simulink model "gm_SuFrame_Scrambler"  (R2023b)
settings: Solver=VariableStepAuto  StartTime=0.0  StopTime=10000/fs  RelTol=1e-3
undefined symbols (not defined in the file or in its folder): fs, iniStates, n, sourceData
libraries: hdlsllib x5, simulink x4
settings Model: Creator=31651  LastModifiedBy=31651
settings OptimizationCC: BlockReduction=off  ConditionallyExecuteInputs=off
settings DebuggingCC: ArtificialAlgebraicLoopMsg=none  InheritedTsInSrcMsg=none

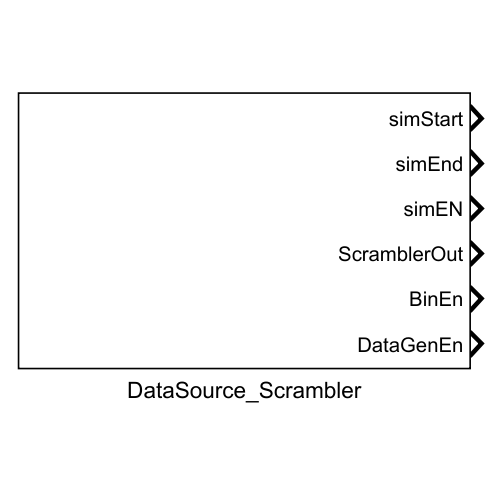
[thumbnail: Simulink's stored preview of the top-level diagram]
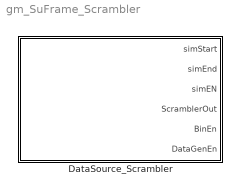
== system gm_SuFrame_Scrambler ==
  DataSource_Scrambler : Subsystem

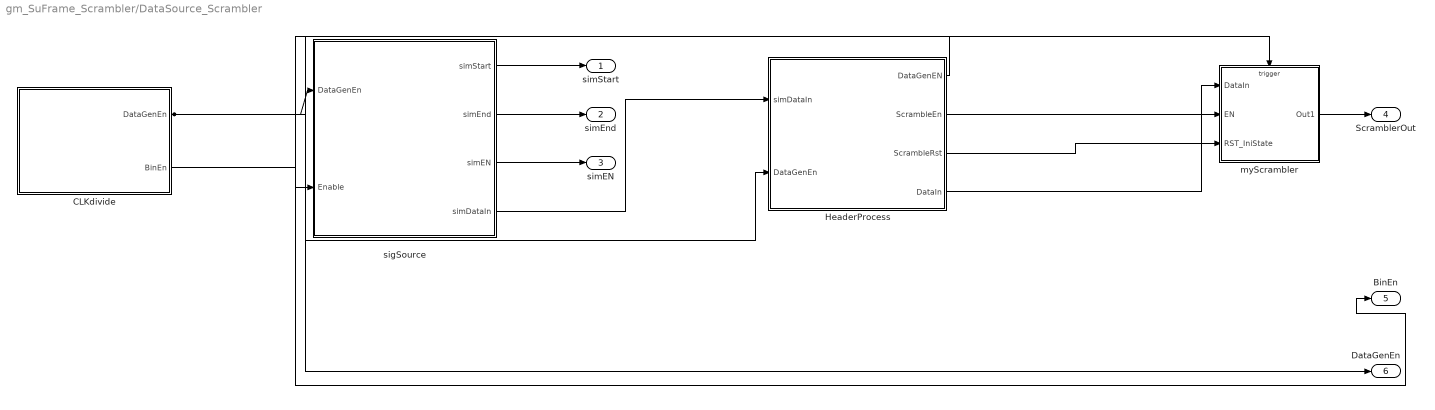
== system gm_SuFrame_Scrambler/DataSource_Scrambler ==
  CLKdivide : Subsystem
  HeaderProcess : Subsystem
  myScrambler : Subsystem
  sigSource : Subsystem
  simStart : Outport  SampleTime=5e-09
  simEnd : Outport  Port=2  SampleTime=5e-09
  simEN : Outport  Port=3  SampleTime=5e-09
  ScramblerOut : Outport  Port=4  SampleTime=5e-09
  BinEn : Outport  Port=5  SampleTime=5e-09  VectorParamsAs1DForOutWhenUnconnected=off
  DataGenEn : Outport  Port=6  SampleTime=5e-09  VectorParamsAs1DForOutWhenUnconnected=off
  wires:
  CLKdivide/1(DataGenEn) -> DataGenEn/1, myScrambler/Trigger, HeaderProcess/2(DataGenEn), sigSource/1(DataGenEn)
  CLKdivide/2(BinEn) -> BinEn/1
  HeaderProcess/2(ScrambleEn) -> myScrambler/2(EN)
  HeaderProcess/3(ScrambleRst) -> myScrambler/3(RST_IniState)
  HeaderProcess/4(DataIn) -> myScrambler/1(DataIn)
  myScrambler/1(Out1) -> ScramblerOut/1
  sigSource/1(simStart) -> simStart/1
  sigSource/2(simEnd) -> simEnd/1
  sigSource/3(simEN) -> simEN/1
  HeaderProcess/1(DataGenEN) -> sigSource/2(Enable)
  sigSource/4(simDataIn) -> HeaderProcess/1(simDataIn)

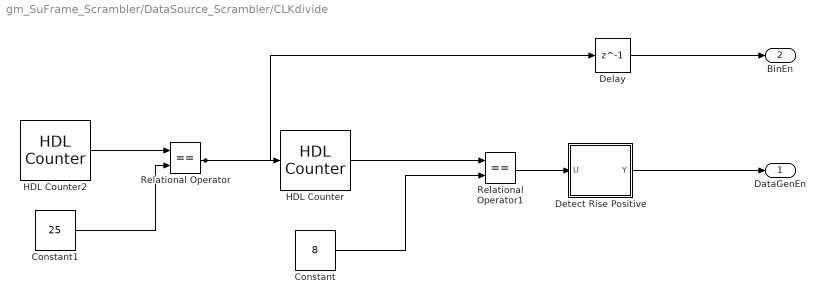
== system gm_SuFrame_Scrambler/DataSource_Scrambler/CLKdivide ==
  Constant : Constant  Value=8  VectorParams1D=off  OutDataTypeStr=uint8  SampleTime=-1
  Constant1 : Constant  Value=25  VectorParams1D=off  OutDataTypeStr=uint8  SampleTime=-1
  Delay : Delay  DelayLength=1
  Detect Rise Positive : Subsystem  mask(Detect Rise Positive){vinit=double(0), InputProcessing=Elements as channels (sample based), OutDataTypeStr=boolean}
      mask prompts: vinit "Simulink:masks:InitialCondition_MP"; InputProcessing "Simulink:masks:InputProcessing_MP"; OutDataTypeStr "Simulink:masks:OutputDataType_MP"
      mask help: Simulink:masks:DetectRisePositive_MD
      mask init:
      | InputProcessing = 'Elements as channels (sample based)';
      | OutDataTypeStr = 'boolean';
      | vinit = double(0);
      mask TypeOptions InputProcessing: Simulink:masks:ColumnsAsChannelsFrameBased | Simulink:masks:ElementsAsChannelsSampleBased
      mask TypeOptions OutDataTypeStr: Simulink:masks:uint8 | Simulink:masks:boolean
      mask Display: fprintf('U > 0\n&  NOT\nU/z > 0')
  HDL Counter : hdlsllib/Sources/HDL Counter  CountType=Count limited  CountInit=1  CountStep=1  CountMax=8  CountFromType=Initial value  CountFrom=1  CountResetPort=off  CountLoadPort=off  CountEnbPort=on  CountDirPort=off  CountHitOutputPort=off  CountDataType=Unsigned  CountWordLen=8  CountFracLen=0  CountSampTime=1
  HDL Counter2 : hdlsllib/Sources/HDL Counter  CountType=Count limited  CountInit=1  CountStep=1  CountMax=25  CountFromType=Initial value  CountFrom=1  CountResetPort=off  CountLoadPort=off  CountEnbPort=off  CountDirPort=off  CountHitOutputPort=off  CountDataType=Unsigned  CountWordLen=8  CountFracLen=0  CountSampTime=1/fs
  Relational Operator : RelationalOperator  Operator===  OutDataTypeStr=boolean  InputSameDT=off
  Relational Operator1 : RelationalOperator  Operator===  OutDataTypeStr=boolean  InputSameDT=off
  DataGenEn : Outport  SampleTime=5e-09  VectorParamsAs1DForOutWhenUnconnected=off
  BinEn : Outport  Port=2  SampleTime=5e-09  VectorParamsAs1DForOutWhenUnconnected=off
  wires:
  Constant/1 -> Relational Operator1/2
  Constant1/1 -> Relational Operator/2
  Delay/1 -> BinEn/1
  Detect Rise Positive/1(Y) -> DataGenEn/1
  HDL Counter/1 -> Relational Operator1/1
  HDL Counter2/1 -> Relational Operator/1
  Relational Operator/1 -> Delay/1, HDL Counter/1
  Relational Operator1/1 -> Detect Rise Positive/1(U)

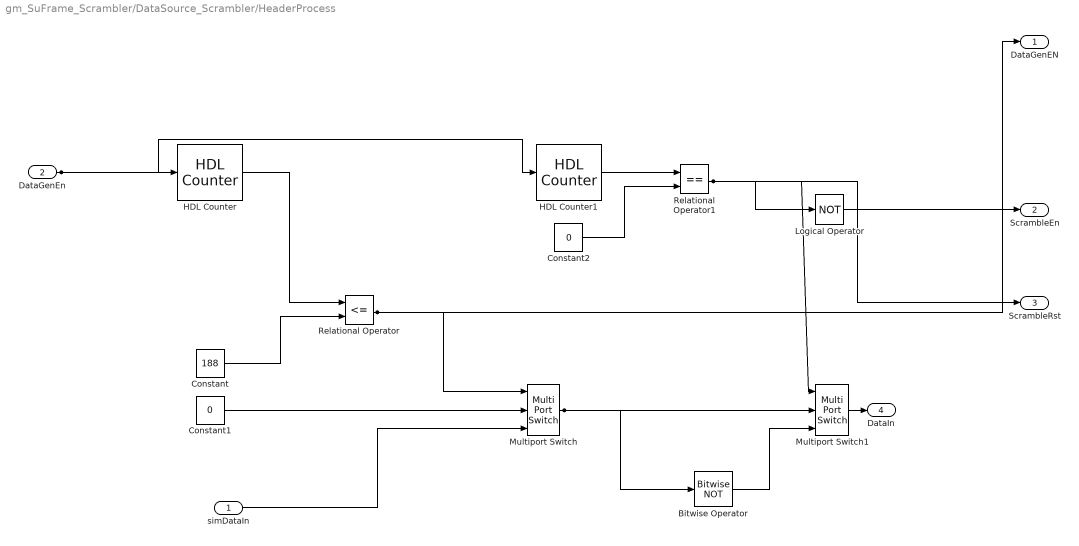
== system gm_SuFrame_Scrambler/DataSource_Scrambler/HeaderProcess ==
  simDataIn : Inport  OutDataTypeStr=uint8  PortDimensions=1  SampleTime=5e-09
  DataGenEn : Inport  Port=2  OutDataTypeStr=boolean  PortDimensions=1  SampleTime=5e-09
  Bitwise Operator : simulink/Logic and Bit Operations/Bitwise Operator  logicop=NOT  UseBitMask=off  BitMask=bin2dec('11011001')  BitMaskRealWorld=Stored Integer
  Constant : Constant  Value=188  OutDataTypeStr=uint8  SampleTime=1/fs
  Constant1 : Constant  Value=0  OutDataTypeStr=uint8
  Constant2 : Constant  Value=0  OutDataTypeStr=uint8
  HDL Counter : hdlsllib/Sources/HDL Counter  CountType=Count limited  CountInit=1  CountStep=1  CountMax=n  CountFromType=Initial value  CountFrom=1  CountResetPort=off  CountLoadPort=off  CountEnbPort=on  CountDirPort=off  CountHitOutputPort=off  CountDataType=Unsigned  CountWordLen=8  CountFracLen=0  CountSampTime=1/fs
  HDL Counter1 : hdlsllib/Sources/HDL Counter  CountType=Count limited  CountInit=0  CountStep=1  CountMax=n*8-1  CountFromType=Initial value  CountFrom=0  CountResetPort=off  CountLoadPort=off  CountEnbPort=on  CountDirPort=off  CountHitOutputPort=off  CountDataType=Unsigned  CountWordLen=16  CountFracLen=0  CountSampTime=1/fs
  Logical Operator : Logic  Operator=NOT  AllPortsSameDT=off  OutDataTypeStr=boolean
  Multiport Switch : MultiPortSwitch  DataPortOrder=Specify indices  DataPortIndices={0,1}  OutDataTypeStr=uint8  SaturateOnIntegerOverflow=off  InputSameDT=off
  Multiport Switch1 : MultiPortSwitch  DataPortOrder=Specify indices  DataPortIndices={0,1}  OutDataTypeStr=uint8  SaturateOnIntegerOverflow=off  InputSameDT=off
  Relational Operator : RelationalOperator  Operator=<=  OutDataTypeStr=boolean  InputSameDT=off
  Relational Operator1 : RelationalOperator  Operator===  OutDataTypeStr=boolean  InputSameDT=off
  DataGenEN : Outport  SampleTime=5e-09  VectorParamsAs1DForOutWhenUnconnected=off
  ScrambleEn : Outport  Port=2  SampleTime=5e-09  VectorParamsAs1DForOutWhenUnconnected=off
  ScrambleRst : Outport  Port=3  SampleTime=5e-09  VectorParamsAs1DForOutWhenUnconnected=off
  DataIn : Outport  Port=4  SampleTime=5e-09
  wires:
  simDataIn/1 -> Multiport Switch/3
  DataGenEn/1 -> HDL Counter/1, HDL Counter1/1
  Bitwise Operator/1 -> Multiport Switch1/3
  Constant/1 -> Relational Operator/2
  Constant1/1 -> Multiport Switch/2
  Constant2/1 -> Relational Operator1/2
  HDL Counter/1 -> Relational Operator/1
  HDL Counter1/1 -> Relational Operator1/1
  Logical Operator/1 -> ScrambleEn/1
  Multiport Switch/1 -> Multiport Switch1/2, Bitwise Operator/1
  Multiport Switch1/1 -> DataIn/1
  Relational Operator/1 -> Multiport Switch/1, DataGenEN/1
  Relational Operator1/1 -> Multiport Switch1/1, Logical Operator/1, ScrambleRst/1

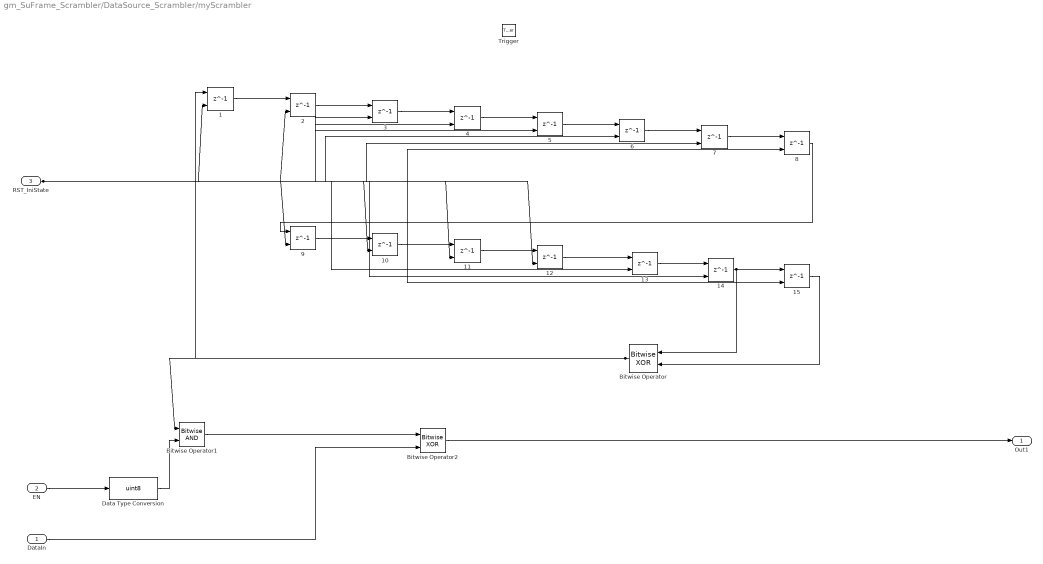
== system gm_SuFrame_Scrambler/DataSource_Scrambler/myScrambler ==
  DataIn : Inport  OutDataTypeStr=uint8  PortDimensions=1
  EN : Inport  Port=2  OutDataTypeStr=boolean  PortDimensions=1
  RST_IniState : Inport  Port=3  OutDataTypeStr=boolean  PortDimensions=1
  Trigger : TriggerPort  VariantControl=(inherit)  PortDimensions=1  OutDataTypeStr=boolean
  1 : Delay  DelayLength=1  InitialCondition=iniStates(1)  ExternalReset=Level
      settings: InputPortMap=u0,r5
  10 : Delay  DelayLength=1  InitialCondition=iniStates(10)  ExternalReset=Level
      settings: InputPortMap=u0,r5
  11 : Delay  DelayLength=1  InitialCondition=iniStates(11)  ExternalReset=Level
      settings: InputPortMap=u0,r5
  12 : Delay  DelayLength=1  InitialCondition=iniStates(12)  ExternalReset=Level
      settings: InputPortMap=u0,r5
  13 : Delay  DelayLength=1  InitialCondition=iniStates(13)  ExternalReset=Level
      settings: InputPortMap=u0,r5
  14 : Delay  DelayLength=1  InitialCondition=iniStates(14)  ExternalReset=Level
      settings: InputPortMap=u0,r5
  15 : Delay  DelayLength=1  InitialCondition=iniStates(15)  ExternalReset=Level
      settings: InputPortMap=u0,r5
  2 : Delay  DelayLength=1  InitialCondition=iniStates(2)  ExternalReset=Level
      settings: InputPortMap=u0,r5
  3 : Delay  DelayLength=1  InitialCondition=iniStates(3)  ExternalReset=Level
      settings: InputPortMap=u0,r5
  4 : Delay  DelayLength=1  InitialCondition=iniStates(4)  ExternalReset=Level
      settings: InputPortMap=u0,r5
  5 : Delay  DelayLength=1  InitialCondition=iniStates(5)  ExternalReset=Level
      settings: InputPortMap=u0,r5
  6 : Delay  DelayLength=1  InitialCondition=iniStates(6)  ExternalReset=Level
      settings: InputPortMap=u0,r5
  7 : Delay  DelayLength=1  InitialCondition=iniStates(7)  ExternalReset=Level
      settings: InputPortMap=u0,r5
  8 : Delay  DelayLength=1  InitialCondition=iniStates(8)  ExternalReset=Level
      settings: InputPortMap=u0,r5
  9 : Delay  DelayLength=1  InitialCondition=iniStates(9)  ExternalReset=Level
      settings: InputPortMap=u0,r5
  Bitwise Operator : simulink/Logic and Bit Operations/Bitwise Operator  logicop=XOR  UseBitMask=off  NumInputPorts=2  BitMask=bin2dec('11011001')  BitMaskRealWorld=Stored Integer
  Bitwise Operator1 : simulink/Logic and Bit Operations/Bitwise Operator  logicop=AND  UseBitMask=off  NumInputPorts=2  BitMask=bin2dec('11011001')  BitMaskRealWorld=Stored Integer
  Bitwise Operator2 : simulink/Logic and Bit Operations/Bitwise Operator  logicop=XOR  UseBitMask=off  NumInputPorts=2  BitMask=bin2dec('11011001')  BitMaskRealWorld=Stored Integer
  Data Type Conversion : DataTypeConversion  OutDataTypeStr=uint8  SaturateOnIntegerOverflow=off  RndMeth=Floor
  Out1 : Outport  InitialOutput=0
  wires:
  DataIn/1 -> Bitwise Operator2/2
  EN/1 -> Data Type Conversion/1
  RST_IniState/1 -> 14/2, 13/2, 12/2, 11/2, 10/2, 9/2, 8/2, 7/2, 6/2, 5/2, 4/2, 3/2, 2/2, 1/2, 15/2
  Bitwise Operator/1 -> Bitwise Operator1/1, 1/1
  Bitwise Operator1/1 -> Bitwise Operator2/1
  Bitwise Operator2/1 -> Out1/1
  Data Type Conversion/1 -> Bitwise Operator1/2
  15/1 -> Bitwise Operator/2
  1/1 -> 2/1
  2/1 -> 3/1
  3/1 -> 4/1
  4/1 -> 5/1
  5/1 -> 6/1
  6/1 -> 7/1
  7/1 -> 8/1
  8/1 -> 9/1
  9/1 -> 10/1
  10/1 -> 11/1
  11/1 -> 12/1
  12/1 -> 13/1
  13/1 -> 14/1
  14/1 -> Bitwise Operator/1, 15/1

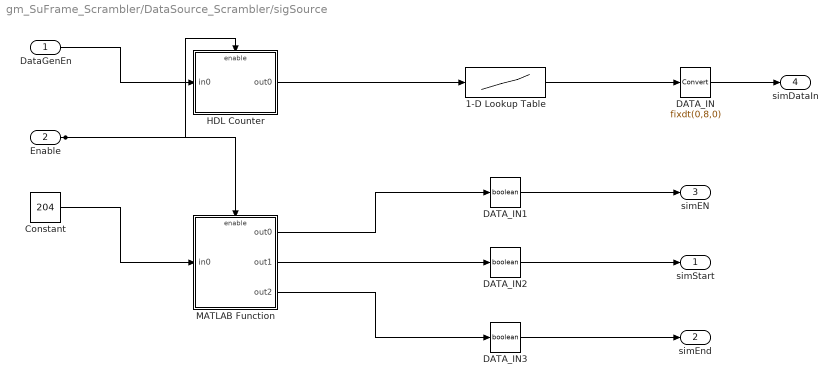
== system gm_SuFrame_Scrambler/DataSource_Scrambler/sigSource ==
  DataGenEn : Inport  OutDataTypeStr=boolean  PortDimensions=1  SampleTime=5e-09
  Enable : Inport  Port=2  OutDataTypeStr=boolean  SampleTime=5e-09
  1-D Lookup Table : Lookup_n-D  NumberOfTableDimensions=1  LookupTableObject=''  BreakpointsForDimension1=[0:18800-1]'  BreakpointsForDimension1FirstPoint=10  BreakpointsForDimension2FirstPoint=10  BreakpointsForDimension1Spacing=12  BreakpointsForDimension2Spacing=12  IndexSearchMethod=Evenly spaced points  Table=sourceData  InterpMethod=Flat  InternalRulePriority=Speed  OutDataTypeStr=uint8  RndMeth=Simplest
  Constant : Constant  Value=204  OutDataTypeStr=uint16  SampleTime=5e-09
  DATA_IN : DataTypeConversion  OutDataTypeStr=fixdt(0,8,0)
  DATA_IN1 : DataTypeConversion  OutDataTypeStr=boolean  SampleTime=5e-09  SaturateOnIntegerOverflow=off  RndMeth=Floor
  DATA_IN2 : DataTypeConversion  OutDataTypeStr=boolean  SampleTime=5e-09  SaturateOnIntegerOverflow=off  RndMeth=Floor
  DATA_IN3 : DataTypeConversion  OutDataTypeStr=boolean  SampleTime=5e-09  SaturateOnIntegerOverflow=off  RndMeth=Floor
  HDL Counter : Subsystem
      settings: MinAlgLoopOccurrences=on
  MATLAB Function : Subsystem
      settings: MinAlgLoopOccurrences=on
  simStart : Outport  SampleTime=5e-09  InitialOutput=0
  simEnd : Outport  Port=2  SampleTime=5e-09  InitialOutput=0
  simEN : Outport  Port=3  SampleTime=5e-09  InitialOutput=0
  simDataIn : Outport  Port=4  SampleTime=5e-09  InitialOutput=0
  wires:
  Enable/1 -> HDL Counter/Enable, MATLAB Function/Enable
  DataGenEn/1 -> HDL Counter/1(in0)
  1-D Lookup Table/1 -> DATA_IN/1
  Constant/1 -> MATLAB Function/1(in0)
  DATA_IN/1 -> simDataIn/1
  DATA_IN1/1 -> simEN/1
  DATA_IN2/1 -> simStart/1
  DATA_IN3/1 -> simEnd/1
  HDL Counter/1(out0) -> 1-D Lookup Table/1
  MATLAB Function/1(out0) -> DATA_IN1/1
  MATLAB Function/2(out1) -> DATA_IN2/1
  MATLAB Function/3(out2) -> DATA_IN3/1

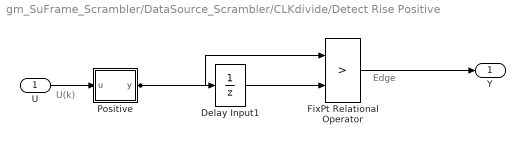
== system gm_SuFrame_Scrambler/DataSource_Scrambler/CLKdivide/Detect Rise Positive ==
  note: Edge
  note: U(k)
  U : Inport  OutDataTypeStr=boolean  SampleTime=5e-09
  Delay Input1 : UnitDelay  Description=Store in Global RAM  DisableCoverage=on  InitialCondition=vinit  SampleTime=-1  HasFrameUpgradeWarning=on
  FixPt Relational Operator : RelationalOperator  Operator=>  OutDataTypeStr=boolean  ZeroCross=off  InputSameDT=off
  Positive : Subsystem  mask(Compare To Zero){relop=>, OutDataTypeStr=boolean, ZeroCross=off}
      mask prompts: relop "Simulink:masks:Operator_MP"; OutDataTypeStr "Simulink:masks:OutputDataType_MP"; ZeroCross "Simulink:masks:EnableZerocrossingDetection_MP"
      mask help: Simulink:masks:CompareToZero_MD
      mask init:
      | OutDataTypeStr = 'boolean';
      | ZeroCross = 'off';
      | blkName = 'SuFrame_Scrambler/DataSource_Scrambler/CLKdivide/Detect Rise\nPositive/Positive';
      | relop = '>';
      | setValue = 'boolean';
      mask TypeOptions relop: == | ~= | < | <= | >= | >
      mask TypeOptions OutDataTypeStr: Simulink:masks:uint8 | Simulink:masks:boolean
      mask Callback ZeroCross: sl('zeroCrossEnable', gcbh);
      mask Display: disp([relop,' 0'])
  Y : Outport  SampleTime=5e-09
  wires:
  U/1 -> Positive/1(u)
  Delay Input1/1 -> FixPt Relational Operator/2
  FixPt Relational Operator/1 -> Y/1
  Positive/1(y) -> FixPt Relational Operator/1, Delay Input1/1

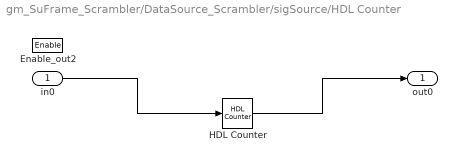
== system gm_SuFrame_Scrambler/DataSource_Scrambler/sigSource/HDL Counter ==
  in0 : Inport  OutDataTypeStr=boolean  SampleTime=5e-09
  Enable_out2 : EnablePort  OutDataTypeStr=boolean
  HDL Counter : hdlsllib/Sources/HDL Counter  CountType=Count limited  CountInit=0  CountStep=1  CountMax=18800-1  CountFromType=Initial value  CountFrom=0  CountResetPort=off  CountLoadPort=off  CountEnbPort=on  CountDirPort=off  CountHitOutputPort=off  CountDataType=Unsigned  CountWordLen=32  CountFracLen=0  CountSampTime=1/fs
  out0 : Outport  OutDataTypeStr=uint32  SampleTime=5e-09  InitialOutput=0
  wires:
  HDL Counter/1 -> out0/1
  in0/1 -> HDL Counter/1

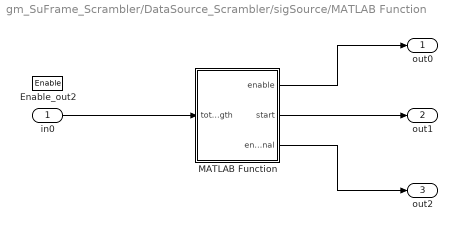
== system gm_SuFrame_Scrambler/DataSource_Scrambler/sigSource/MATLAB Function ==
  in0 : Inport  OutDataTypeStr=uint16  SampleTime=5e-09
  Enable_out2 : EnablePort  OutDataTypeStr=boolean
  MATLAB Function : Subsystem
  out0 : Outport  OutDataTypeStr=uint8  SampleTime=5e-09  InitialOutput=0
  out1 : Outport  Port=2  OutDataTypeStr=uint8  SampleTime=5e-09  InitialOutput=0
  out2 : Outport  Port=3  OutDataTypeStr=uint8  SampleTime=5e-09  InitialOutput=0
  wires:
  MATLAB Function/1(enable) -> out0/1
  MATLAB Function/2(start) -> out1/1
  MATLAB Function/3(endSignal) -> out2/1
  in0/1 -> MATLAB Function/1(totalLength)

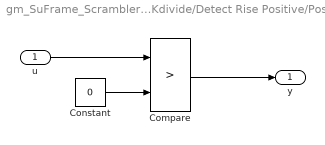
== system gm_SuFrame_Scrambler/DataSource_Scrambler/CLKdivide/Detect Rise Positive/Positive ==
  u : Inport  OutDataTypeStr=boolean  SampleTime=5e-09
  Compare : RelationalOperator  Operator=>  OutDataTypeStr=boolean  ZeroCross=off
  Constant : Constant  DisableCoverage=on  Value=0  OutDataTypeStr=Inherit: Inherit via back propagation  SampleTime=-1  PreserveConstantTs=on
  y : Outport  SampleTime=5e-09
  wires:
  u/1 -> Compare/1
  Compare/1 -> y/1
  Constant/1 -> Compare/2

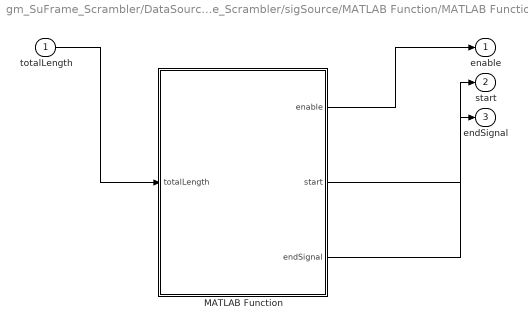
== system gm_SuFrame_Scrambler/DataSource_Scrambler/sigSource/MATLAB Function/MATLAB Function ==
  totalLength : Inport  OutDataTypeStr=uint16  PortDimensions=1  SampleTime=5e-09
  MATLAB Function : MATLAB Function  TreatAsAtomicUnit=on
  enable : Outport  SampleTime=5e-09  InitialOutput=0  VectorParamsAs1DForOutWhenUnconnected=off
  start : Outport  Port=2  SampleTime=5e-09  InitialOutput=0
  endSignal : Outport  Port=3  SampleTime=5e-09  InitialOutput=0
  wires:
  MATLAB Function/1(enable) -> enable/1
  MATLAB Function/2(start) -> start/1
  MATLAB Function/3(endSignal) -> endSignal/1
  totalLength/1 -> MATLAB Function/1(totalLength)

== matlab function gm_SuFrame_Scrambler/DataSource_Scrambler/sigSource/MATLAB Function/MATLAB Function/MATLAB Function ==
  data: totalLength input; enable output; start output; endSignal output
function [enable, start, endSignal] = rsSignals(totalLength)
    % rsSignals Generate enable, start, and end signals for RS(188,204)
    %
    % Input:
    %   totalLength - Total number of cycles the signals are active
    %
    % Output:
    %   enable - Enable signal (1 during transmission, 0 otherwise) as uint8
    %   start - Start signal (1 at the first cycle, 0 otherwise) as uint8
    %   endSignal - End signal (1 at the last cycle, 0 otherwise) as uint8

    % Persistent variable to keep track of the current cycle, as uint8
    persistent cycle;
    if isempty(cycle)
        cycle = uint8(0);  % Initialize the cycle count
    end

    % Increment cycle count
    cycle = cycle + 1;

    % Generate start signal
    if cycle == 1
        start = uint8(1);
    else
        start = uint8(0);
    end

    % Generate enable signal
    if cycle > 0 && cycle <= totalLength
        enable = uint8(1);
    else
        enable = uint8(0);
    end

    % Generate end signal
    if cycle == 188
        endSignal = uint8(1);
    else
        endSignal = uint8(0);
    end

    % Reset cycle count after reaching total length
    if cycle >= totalLength
        cycle = uint8(0);
    end
end
